simulink model "EKF_KTeam"  (R2014a)
settings: Solver=ode45  StartTime=0.0  StopTime=380  RelTol=1e-3
libraries: simulink x6
settings Model: Creator=KTeamRoot  LastModifiedBy=Bird
settings DebuggingCC: UnderspecifiedInitializationDetection=Classic  StateNameClashWarn=warning

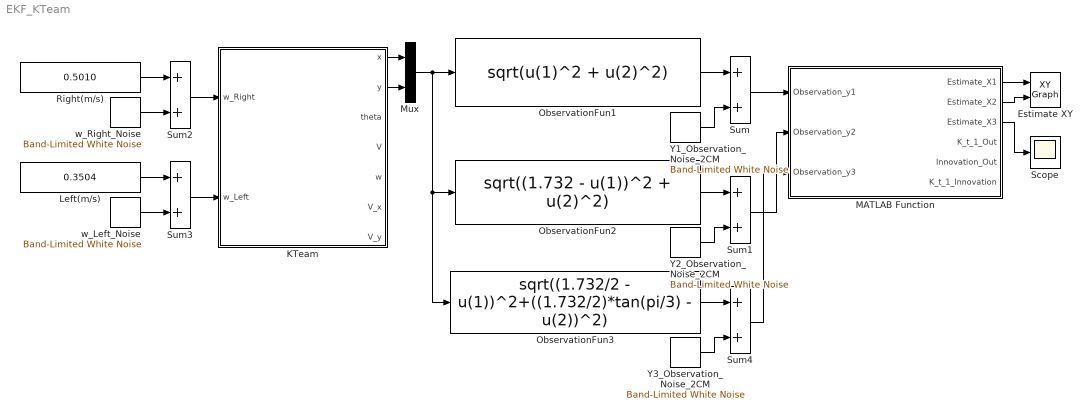
== system EKF_KTeam ==
  Estimate XY : simulink/Sinks/XY Graph  xmin=-0.5  xmax=1.732  ymin=-0.5  ymax=1.5  st=-1
  KTeam : Subsystem  mask(KTeamRobot){wRightLimit=3.33522405, wLeftLimit=3.33522405, w_Right_ACCLimit=3.33522405/0.5, w_Left_ACCLimit=3.33522405/0.5, Right_Radius=41/2, Left_Radius=41/2, b=88.41, KTeamSampleTime=0.1, handbrake=0, x0=0, x1=1.732/2, x2=0.25}
      mask prompts: wRightLimit "右轮速度极限(rad/s)"; wLeftLimit "左轮速度极限(rad/s)"; w_Right_ACCLimit "右轮加速度极限(rad/s2)"; w_Left_ACCLimit "左轮加速度极限(rad/s2)"; Right_Radius "右轮半径(mm)"; Left_Radius "左轮半径(mm)"; b "两轮轴距(mm)"; KTeamSampleTime "采样时间(s)"; handbrake "脚刹车"; x0 "机器人角度初始值(m)"; x1 "机器人初始X坐标(m)"; x2 "机器人初始Y坐标(m)"
      mask help: 这个模块模拟KTeam机器人
      mask Display:
      | disp('KTeamRobot');
      | port_label('output', 1, 'x');
      | port_label('output', 2, 'y');
      | port_label('output', 3, 'theta');
      | port_label('output', 4, 'v');
      | port_label('output', 5, 'w');
      | port_label('output', 6, 'V_x');
      | port_label('output', 7, 'V_y');
      | port_label('input', 1, 'w_Right');
      | port_label('input', 2, 'w_Left');
  Left(m/s) : Constant  Value=0.3504
  MATLAB Function : MATLAB Function  TreatAsAtomicUnit=on
  Mux : Mux  Inputs=2
  ObservationFun1 : Fcn  Expr=sqrt(u(1)^2 + u(2)^2)
  ObservationFun2 : Fcn  Expr=sqrt((1.732 - u(1))^2 + u(2)^2)
  ObservationFun3 : Fcn  Expr=sqrt((1.732/2 - u(1))^2+((1.732/2)*tan(pi/3) - u(2))^2)
  Right(m/s) : Constant  Value=0.5010
  Scope : Scope
  Sum : Sum  SampleTime=0.4
  Sum1 : Sum  SampleTime=0.4
  Sum2 : Sum
  Sum3 : Sum
  Sum4 : Sum  SampleTime=0.4
  Y1_Observation_Noise_2CM : simulink/Sources/Band-Limited White Noise  Cov=[(0.333e-2)^2*(2*pi/(100*5))]  Ts=2*pi/(100*5)  seed=[17432]
  Y2_Observation_Noise_2CM : simulink/Sources/Band-Limited White Noise  Cov=[(0.333e-2)^2*(2*pi/(100*5))]  Ts=2*pi/(100*5)  seed=[30589]
  Y3_Observation_Noise_2CM : simulink/Sources/Band-Limited White Noise  Cov=[(0.333e-2)^2*(2*pi/(100*5))]  Ts=2*pi/(100*5)  seed=[30589]
  w_Left_Noise : simulink/Sources/Band-Limited White Noise  Cov=[(8*pi/4198)^2*(2*pi/(100*5))]  Ts=2*pi/(100*5)  seed=[38420]
  w_Right_Noise : simulink/Sources/Band-Limited White Noise  Cov=[(8*pi/4198)^2*(2*pi/(100*5))]  Ts=2*pi/(100*5)  seed=[23767]
  wires:
  Y1_Observation_Noise_2CM/1 -> Sum/2
  Y2_Observation_Noise_2CM/1 -> Sum1/2
  w_Right_Noise/1 -> Sum2/2
  w_Left_Noise/1 -> Sum3/2
  Right(m/s)/1 -> Sum2/1
  Left(m/s)/1 -> Sum3/1
  Sum2/1 -> KTeam/1(w_Right)
  Sum3/1 -> KTeam/2(w_Left)
  KTeam/1(x) -> Mux/1
  KTeam/2(y) -> Mux/2
  Mux/1 -> ObservationFun3/1, ObservationFun2/1, ObservationFun1/1
  ObservationFun1/1 -> Sum/1
  ObservationFun2/1 -> Sum1/1
  Y3_Observation_Noise_2CM/1 -> Sum4/2
  ObservationFun3/1 -> Sum4/1
  Sum/1 -> MATLAB Function/1(Observation_y1)
  Sum1/1 -> MATLAB Function/2(Observation_y2)
  Sum4/1 -> MATLAB Function/3(Observation_y3)
  MATLAB Function/1(Estimate_X1) -> Estimate XY/1
  MATLAB Function/2(Estimate_X2) -> Estimate XY/2
  MATLAB Function/3(Estimate_X3) -> Scope/1

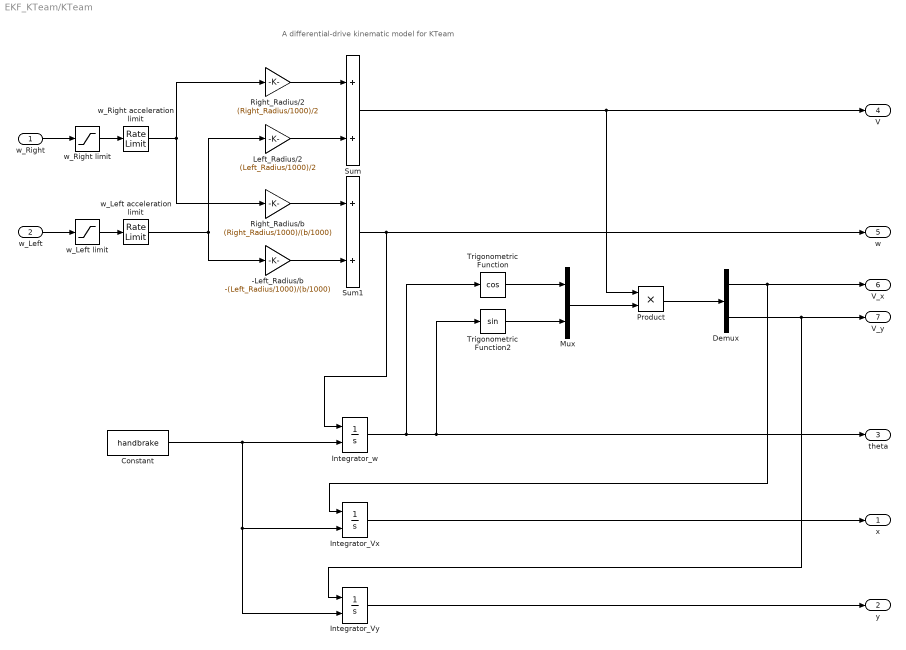
== system EKF_KTeam/KTeam ==
  note: A differential-drive kinematic model for KTeam
  w_Right : Inport
  w_Left : Inport  Port=2
  -Left_Radius/b : Gain  Gain=-(Left_Radius/1000)/(b/1000)
  Constant : Constant  Value=handbrake
  Demux : Demux  Outputs=2
  Integrator_Vx : Integrator  ExternalReset=level  InitialCondition=x1
  Integrator_Vy : Integrator  ExternalReset=level  InitialCondition=x2
  Integrator_w : Integrator  ExternalReset=level  InitialCondition=x0
  Left_Radius/2 : Gain  Gain=(Left_Radius/1000)/2
  Mux : Mux  Inputs=2
  Product : Product  RndMeth=Zero
  Right_Radius/2 : Gain  Gain=(Right_Radius/1000)/2
  Right_Radius/b : Gain  Gain=(Right_Radius/1000)/(b/1000)
  Sum : Sum
  Sum1 : Sum
  Trigonometric Function : Trigonometry  Operator=cos
  Trigonometric Function2 : Trigonometry
  w_Left acceleration limit : RateLimiter  RisingSlewLimit=w_Left_ACCLimit  FallingSlewLimit=-w_Left_ACCLimit  SampleTimeMode=inherited
  w_Left limit : Saturate  UpperLimit=wLeftLimit  LowerLimit=-wLeftLimit  SampleTime=KTeamSampleTime
  w_Right acceleration limit : RateLimiter  RisingSlewLimit=w_Right_ACCLimit  FallingSlewLimit=-w_Right_ACCLimit  SampleTimeMode=inherited
  w_Right limit : Saturate  UpperLimit=wRightLimit  LowerLimit=-wRightLimit  SampleTime=KTeamSampleTime
  x : Outport
  y : Outport  Port=2
  theta : Outport  Port=3
  V : Outport  Port=4
  w : Outport  Port=5
  V_x : Outport  Port=6
  V_y : Outport  Port=7
  wires:
  Integrator_Vx/1 -> x/1
  Integrator_Vy/1 -> y/1
  w_Left limit/1 -> w_Left acceleration limit/1
  Sum/1 -> V/1, Product/1
  w_Right acceleration limit/1 -> Right_Radius/b/1, Right_Radius/2/1
  w_Left acceleration limit/1 -> -Left_Radius/b/1, Left_Radius/2/1
  Demux/1 -> V_x/1, Integrator_Vx/1
  Demux/2 -> V_y/1, Integrator_Vy/1
  Product/1 -> Demux/1
  w_Right/1 -> w_Right limit/1
  w_Right limit/1 -> w_Right acceleration limit/1
  Left_Radius/2/1 -> Sum/2
  w_Left/1 -> w_Left limit/1
  Right_Radius/2/1 -> Sum/1
  Mux/1 -> Product/2
  Trigonometric Function/1 -> Mux/1
  Integrator_w/1 -> Trigonometric Function/1, theta/1, Trigonometric Function2/1
  Trigonometric Function2/1 -> Mux/2
  Right_Radius/b/1 -> Sum1/1
  -Left_Radius/b/1 -> Sum1/2
  Constant/1 -> Integrator_w/2, Integrator_Vy/2, Integrator_Vx/2
  Sum1/1 -> w/1, Integrator_w/1

== matlab function EKF_KTeam/MATLAB Function ==
  data: Observation_y1 input; Observation_y2 input; Observation_y3 input; Estimate_X1 output; Estimate_X2 output; Estimate_X3 output; K_t_1_Out output; Innovation_Out output; K_t_1_Innovation output
function [Estimate_X1,Estimate_X2,Estimate_X3,K_t_1_Out,Innovation_Out,K_t_1_Innovation] = EKF(Observation_y1,Observation_y2,Observation_y3)
%#codegen
%% 基本参数设定%
T = 0.1; %SampleTime
KTeam_Radius_Right = 41/2/1000;
KTeam_Radius_Left = 41/2/1000; %轮子半径

KTeam_WheelBase = 88.41/1000; %轮子轴距


%% 时标计数,从0开始
persistent TimeCounter_K
if isempty(TimeCounter_K)
    TimeCounter_K = -1;
end
TimeCounter_K = TimeCounter_K + 1;

%% 下面是滤波器过程
Power_Q = diag([(8*pi/4198)^2 (8*pi/4198)^2 (8*pi/4198)^2]);
%Power_Q = diag([0 0]);
%Power_R = diag([(2e-2)^2 (2e-2)^2 (2e-2)^2]);
Power_R = diag([(0.333e-2)^2 (0.333e-2)^2 (0.333e-2)^2]);
StateNumber = 3;

%运行变量
persistent X_t_1_t_1
persistent X_t_1_t;
persistent Innovation;
persistent P_t_1_t;
persistent K_t_1;
persistent P_t_1_t_1;

if isempty(X_t_1_t_1)
    X_t_1_t_1 = [0 0 0]';
    X_t_1_t = [0 0 0]';
    Innovation = [0 0 0]';
    P_t_1_t = zeros(StateNumber,StateNumber);
    K_t_1 = zeros(StateNumber,3);
    P_t_1_t_1 = zeros(StateNumber,StateNumber);
    
end

 %第一步，读取测量值
 y_t_1 = [Observation_y1 Observation_y2 Observation_y3]';
 
 %第二步，计算一步预测
 X_t_1_t = NonlinearSYSModel(X_t_1_t_1(1,1),X_t_1_t_1(2,1),X_t_1_t_1(3,1));
 
 %第三步，计算预报误差的方差
 P_t_1_t = Phi_k(X_t_1_t_1(1,1),X_t_1_t_1(2,1),X_t_1_t_1(3,1)) * P_t_1_t_1 * (Phi_k(X_t_1_t_1(1,1),X_t_1_t_1(2,1),X_t_1_t_1(3,1)))' + Gamma_k(X_t_1_t_1(1,1),X_t_1_t_1(2,1),X_t_1_t_1(3,1)) * Power_Q * (Gamma_k(X_t_1_t_1(1,1),X_t_1_t_1(2,1),X_t_1_t_1(3,1)))';

 %第四步,计算滤波器增益
 K_t_1 = P_t_1_t * (Eta_k(X_t_1_t(1,1),X_t_1_t(2,1),X_t_1_t(3,1)))' * inv((Eta_k(X_t_1_t(1,1),X_t_1_t(2,1),X_t_1_t(3,1))) * P_t_1_t * (Eta_k(X_t_1_t(1,1),X_t_1_t(2,1),X_t_1_t(3,1)))' + Power_R);
 
 %第五步，更新滤波误差的方差
 P_t_1_t_1 = (eye(StateNumber) - K_t_1*(Eta_k(X_t_1_t(1,1),X_t_1_t(2,1),X_t_1_t(3,1)))) * P_t_1_t;
 
 %第六步，计算新息
 Innovation = y_t_1 - NonlinearObservationModel(X_t_1_t(1,1),X_t_1_t(2,1),X_t_1_t(3,1));

 %第七步，输出滤波
 X_t_1_t_1 = X_t_1_t + K_t_1 * Innovation;
 
 K_t_1_Out = K_t_1;
 Innovation_Out = Innovation;
 K_t_1_Innovation = K_t_1 * Innovation;
 
 Estimate_X1 = X_t_1_t_1(1,1);
 Estimate_X2 = X_t_1_t_1(2,1);
 Estimate_X3 = X_t_1_t_1(3,1);


end

%现在写入非线性系统方程
function [NonlinearSYSModel_Out] = NonlinearSYSModel(NonlinearModel_X_k , NonlinearModel_Y_k , NonlinearModel_Theta_k)

 F1 = NonlinearModel_X_k + (4024549212991305*cos(NonlinearModel_Theta_k + 8052063253416397/1152921504606846976))/1152921504606846976;
 F2 = NonlinearModel_Y_k + (4024549212991305*sin(NonlinearModel_Theta_k + 8052063253416397/1152921504606846976))/1152921504606846976;
 F3 = NonlinearModel_Theta_k + 8052063253416397/576460752303423488;

 NonlinearSYSModel_Out = [F1 ; F2 ; F3];
end

function [DiffSYSModel_Out] = Phi_k(NonlinearModel_X_k , NonlinearModel_Y_k , NonlinearModel_Theta_k)

DiffSYSModel_Out = [ 1, 0, -(4024549212991305*sin(NonlinearModel_Theta_k + 8052063253416397/1152921504606846976))/1152921504606846976 ;
 0, 1,  (4024549212991305*cos(NonlinearModel_Theta_k + 8052063253416397/1152921504606846976))/1152921504606846976 ;
 0, 0,                                                                                                          1];
 
end

%现在写入非线性观测方程
function [NonlinearObservationModel_Out] = NonlinearObservationModel(NonlinearModel_X_k , NonlinearModel_Y_k , NonlinearModel_Theta_k)
 F1 = (NonlinearModel_X_k^2 + NonlinearModel_Y_k^2)^(1/2);
 F2 = ((NonlinearModel_X_k - 433/250)^2 + NonlinearModel_Y_k^2)^(1/2);
 F3 = ((NonlinearModel_X_k - 433/500)^2 + (NonlinearModel_Y_k - 6755201279765729/4503599627370496)^2)^(1/2);
 NonlinearObservationModel_Out = [F1 ; F2 ; F3];
end

function [DiffObservationModel_Out] = Eta_k(NonlinearModel_X_k , NonlinearModel_Y_k , NonlinearModel_Theta_k)
DiffObservationModel_Out = [NonlinearModel_X_k/(NonlinearModel_X_k^2 + NonlinearModel_Y_k^2)^(1/2),NonlinearModel_Y_k/(NonlinearModel_X_k^2 + NonlinearModel_Y_k^2)^(1/2), 0;
(2*NonlinearModel_X_k - 433/125)/(2*((NonlinearModel_X_k - 433/250)^2 + NonlinearModel_Y_k^2)^(1/2)),NonlinearModel_Y_k/((NonlinearModel_X_k - 433/250)^2 + NonlinearModel_Y_k^2)^(1/2), 0;
(2*NonlinearModel_X_k - 433/250)/(2*((NonlinearModel_X_k - 433/500)^2 + (NonlinearModel_Y_k - 6755201279765729/4503599627370496)^2)^(1/2)), (2*NonlinearModel_Y_k - 6755201279765729/2251799813685248)/(2*((NonlinearModel_X_k - 433/500)^2 + (NonlinearModel_Y_k - 6755201279765729/4503599627370496)^2)^(1/2)), 0];

 end

function [Gamma_k_Out] = Gamma_k(NonlinearModel_X_k , NonlinearModel_Y_k , NonlinearModel_Theta_k)
 Gamma_k_Out = eye(3);
end
